simulink model "ROBOTIC_ARM_sim_v0"  (R2024b)
settings: Solver=VariableStepAuto  StartTime=0.0  StopTime=5  RelTol=1e-3
model workspace: external: MATLAB File D:\Vaults\Mechatronic Systems Design Project\Arm\Control\robotic_arm_4dof_matlab\scripts\initalize_model.m (data not in the file)
undefined symbols (not defined in the file): cubes, sim_relative, smiData, v_b, X, Y, Z
libraries: sm_lib x75, nesl_utility x21
(part 1 of 2)
settings Model: Creator=Mohammed Hany  LastModifiedBy=Mohammed Hany

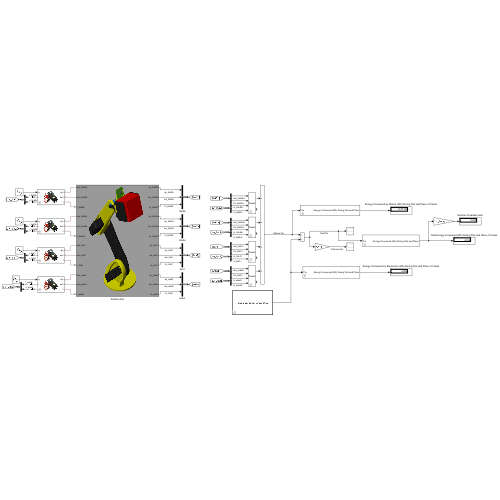
[thumbnail: Simulink's stored preview of the top-level diagram]
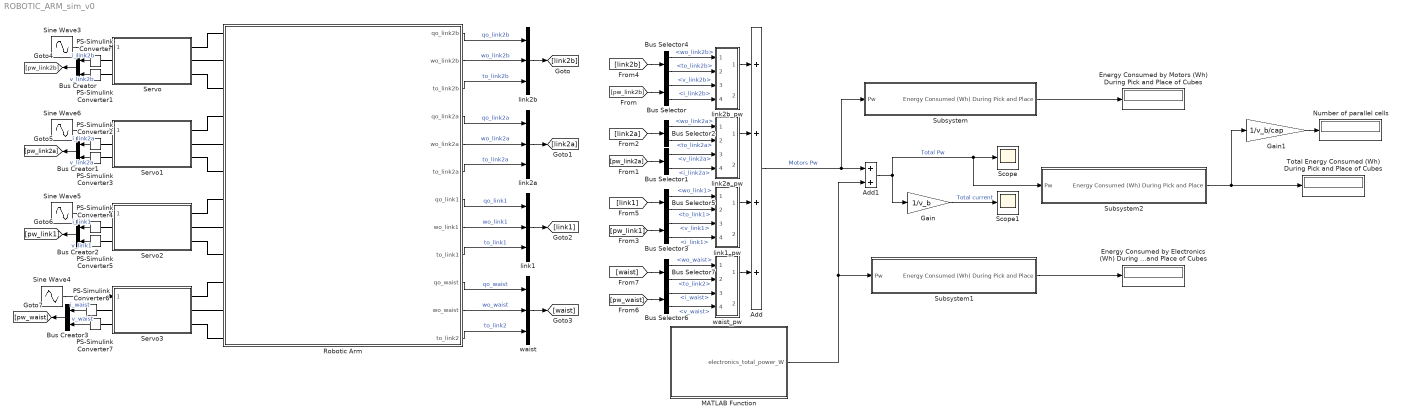
== system ROBOTIC_ARM_sim_v0 ==
  Add : Sum  Inputs=++++
  Add1 : Sum
  Bus Creator{,1..3} (4 alike) : BusCreator  Inputs=2
  Bus Selector : BusSelector  OutputSignals=v_link2b,i_link2b
  Bus Selector1 : BusSelector  OutputSignals=v_link2a,i_link2a
  Bus Selector2 : BusSelector  OutputSignals=wo_link2a,to_link2a
  Bus Selector3 : BusSelector  OutputSignals=v_link1,i_link1
  Bus Selector4 : BusSelector  OutputSignals=wo_link2b,to_link2b
  Bus Selector5 : BusSelector  OutputSignals=wo_link1,to_link1
  Bus Selector6 : BusSelector  OutputSignals=i_waist,v_waist
  Bus Selector7 : BusSelector  OutputSignals=wo_waist,to_link2
  Energy Consumed by Electronics (Wh) During Pick and Place of Cubes : Display
  Energy Consumed by Motors (Wh) During Pick and Place of Cubes : Display
  Gain : Gain  Gain=1/v_b
  Gain1 : Gain  Gain=1/v_b/cap
  MATLAB Function : MATLAB Function  TreatAsAtomicUnit=on
  Number of parallel cells : Display
  PS-Simulink Converter{,2,4,6} (4 alike) : nesl_utility/PS-Simulink Converter  PhysicalDomain=network_engine_domain  SubClassName=ps_output  LeftPortType=input  RightPortType=output  PseudoPeriodic=off  Frequencies=[]  VectorFormat=inherit  Unit=A  AffineConversion=off
  PS-Simulink Converter{1,3,5,7} (4 alike) : nesl_utility/PS-Simulink Converter  PhysicalDomain=network_engine_domain  SubClassName=ps_output  LeftPortType=input  RightPortType=output  PseudoPeriodic=off  Frequencies=[]  VectorFormat=inherit  Unit=V  AffineConversion=off
  Robotic Arm : Subsystem
      mask Display: image('isometric.png');
  Scope : Scope
  Scope1 : Scope
  Servo{,1..3} (4 alike) : Subsystem  ReferencedSubsystem=Servo  J=0 cm^2*g  La=12e-6 H  P_rated=4.2 W  V_i_noload=6 V  V_rated=6 V  i_noload=0.05 A  w_max=99 rpm  w_rated=71.43 rpm  ratio=1
  Sine Wave3 : Sin  Amplitude=55  Bias=30  SampleTime=0
  Sine Wave4 : Sin  Amplitude=180  SampleTime=0
  Sine Wave5 : Sin  Amplitude=100  Bias=-50  SampleTime=0
  Sine Wave6 : Sin  Amplitude=100  Bias=50  SampleTime=0
  Subsystem : Subsystem  mask{cubes=cubes}
      mask prompts: cubes "Number of cubes for pick and place"
  Subsystem1 : Subsystem  mask{cubes=cubes}
      mask prompts: cubes "Number of cubes for pick and place"
  Subsystem2 : Subsystem  mask{cubes=cubes}
      mask prompts: cubes "Number of cubes for pick and place"
  Total Energy Consumed (Wh) During Pick and Place of Cubes : Display
  link1 : BusCreator  Inputs=3
  link1_pw : Subsystem  ReferencedSubsystem=joint_power
  link2a : BusCreator  Inputs=3
  link2a_pw : Subsystem  ReferencedSubsystem=joint_power
  link2b : BusCreator  Inputs=3
  link2b_pw : Subsystem  ReferencedSubsystem=joint_power
  waist : BusCreator  Inputs=3
  waist_pw : Subsystem  ReferencedSubsystem=joint_power
  wires:
  Add/1 -> Subsystem/1(Pw), Add1/1  "Motors Pw"
  Subsystem1/1(Energy Consumed (Wh) During Pick and Place) -> Energy Consumed by Electronics (Wh) During Pick and Place of Cubes/1
  MATLAB Function/1(electronics_total_power_W) -> Add1/2, Subsystem1/1(Pw)
  Subsystem/1(Energy Consumed (Wh) During Pick and Place) -> Energy Consumed by Motors (Wh) During Pick and Place of Cubes/1
  Gain/1 -> Scope1/1  "Total current"
  Add1/1 -> Gain/1, Subsystem2/1(Pw), Scope/1  "Total Pw"
  Subsystem2/1(Energy Consumed (Wh) During Pick and Place) -> Gain1/1, Total Energy Consumed (Wh) During Pick and Place of Cubes/1
  Gain1/1 -> Number of parallel cells/1
  Sine Wave3/1 -> Servo/1
  Sine Wave6/1 -> Servo1/1
  Sine Wave5/1 -> Servo2/1
  Sine Wave4/1 -> Servo3/1
  Robotic Arm/3(to_link2b) -> link2b/3  "to_link2b"
  Robotic Arm/2(wo_link2b) -> link2b/2  "wo_link2b"
  Robotic Arm/1(qo_link2b) -> link2b/1  "qo_link2b"
  Robotic Arm/5(wo_link2a) -> link2a/2  "wo_link2a"
  Robotic Arm/4(qo_link2a) -> link2a/1  "qo_link2a"
  Robotic Arm/6(to_link2a) -> link2a/3  "to_link2a"
  Robotic Arm/8(wo_link1) -> link1/2  "wo_link1"
  Robotic Arm/7(qo_link1) -> link1/1  "qo_link1"
  Robotic Arm/9(to_link1) -> link1/3  "to_link1"
  Robotic Arm/11(wo_waist) -> waist/2  "wo_waist"
  Robotic Arm/10(qo_waist) -> waist/1  "qo_waist"
  Robotic Arm/12(to_link2) -> waist/3  "to_link2"
  link2b/1 -> [link2b]
  link2a/1 -> [link2a]
  link1/1 -> [link1]
  waist/1 -> [waist]
  PS-Simulink Converter/1 -> Bus Creator/1  "i_link2b"
  PS-Simulink Converter1/1 -> Bus Creator/2  "v_link2b"
  Bus Creator/1 -> [pw_link2b]
  PS-Simulink Converter3/1 -> Bus Creator1/2  "v_link2a"
  Bus Creator1/1 -> [pw_link2a]
  PS-Simulink Converter2/1 -> Bus Creator1/1  "i_link2a"
  PS-Simulink Converter4/1 -> Bus Creator2/1  "i_link1"
  PS-Simulink Converter5/1 -> Bus Creator2/2  "v_link1"
  Bus Creator2/1 -> [pw_link1]
  Bus Creator3/1 -> [pw_waist]
  PS-Simulink Converter7/1 -> Bus Creator3/2  "v_waist"
  PS-Simulink Converter6/1 -> Bus Creator3/1  "i_waist"
  [pw_link2b] -> Bus Selector/1
  link2b_pw/1 -> Add/1
  Bus Selector/1 -> link2b_pw/3  "<v_link2b>"
  Bus Selector/2 -> link2b_pw/4  "<i_link2b>"
  [link2b] -> Bus Selector4/1
  Bus Selector4/2 -> link2b_pw/2  "<to_link2b>"
  Bus Selector4/1 -> link2b_pw/1  "<wo_link2b>"
  [link2a] -> Bus Selector2/1
  [pw_link2a] -> Bus Selector1/1
  link2a_pw/1 -> Add/2
  Bus Selector2/1 -> link2a_pw/1  "<wo_link2a>"
  Bus Selector2/2 -> link2a_pw/2  "<to_link2a>"
  [link1] -> Bus Selector5/1
  [pw_link1] -> Bus Selector3/1
  link1_pw/1 -> Add/3
  Bus Selector1/1 -> link2a_pw/3  "<v_link2a>"
  Bus Selector1/2 -> link2a_pw/4  "<i_link2a>"
  Bus Selector5/1 -> link1_pw/1  "<wo_link1>"
  Bus Selector5/2 -> link1_pw/2  "<to_link1>"
  Bus Selector3/1 -> link1_pw/3  "<v_link1>"
  Bus Selector3/2 -> link1_pw/4  "<i_link1>"
  [pw_waist] -> Bus Selector6/1
  [waist] -> Bus Selector7/1
  waist_pw/1 -> Add/4
  Bus Selector7/1 -> waist_pw/1  "<wo_waist>"
  Bus Selector7/2 -> waist_pw/2  "<to_link2>"
  Bus Selector6/1 -> waist_pw/3  "<i_waist>"
  Bus Selector6/2 -> waist_pw/4  "<v_waist>"
  connections:
  Robotic Arm/LConn1 -- Servo/RConn1
  Robotic Arm/LConn2 -- Servo/RConn2
  Robotic Arm/LConn3 -- Servo/RConn3
  Servo1/RConn1 -- Robotic Arm/LConn4
  Robotic Arm/LConn5 -- Servo1/RConn2
  Robotic Arm/LConn6 -- Servo1/RConn3
  Robotic Arm/LConn7 -- Servo2/RConn1
  Robotic Arm/LConn8 -- Servo2/RConn2
  Robotic Arm/LConn9 -- Servo2/RConn3
  Robotic Arm/LConn10 -- Servo3/RConn1
  Robotic Arm/LConn11 -- Servo3/RConn2
  Robotic Arm/LConn12 -- Servo3/RConn3
  Servo/LConn1 -- PS-Simulink Converter/LConn1
  PS-Simulink Converter1/LConn1 -- Servo/LConn2
  Servo1/LConn1 -- PS-Simulink Converter2/LConn1
  Servo1/LConn2 -- PS-Simulink Converter3/LConn1
  Servo2/LConn1 -- PS-Simulink Converter4/LConn1
  Servo2/LConn2 -- PS-Simulink Converter5/LConn1
  Servo3/LConn1 -- PS-Simulink Converter6/LConn1
  PS-Simulink Converter7/LConn1 -- Servo3/LConn2

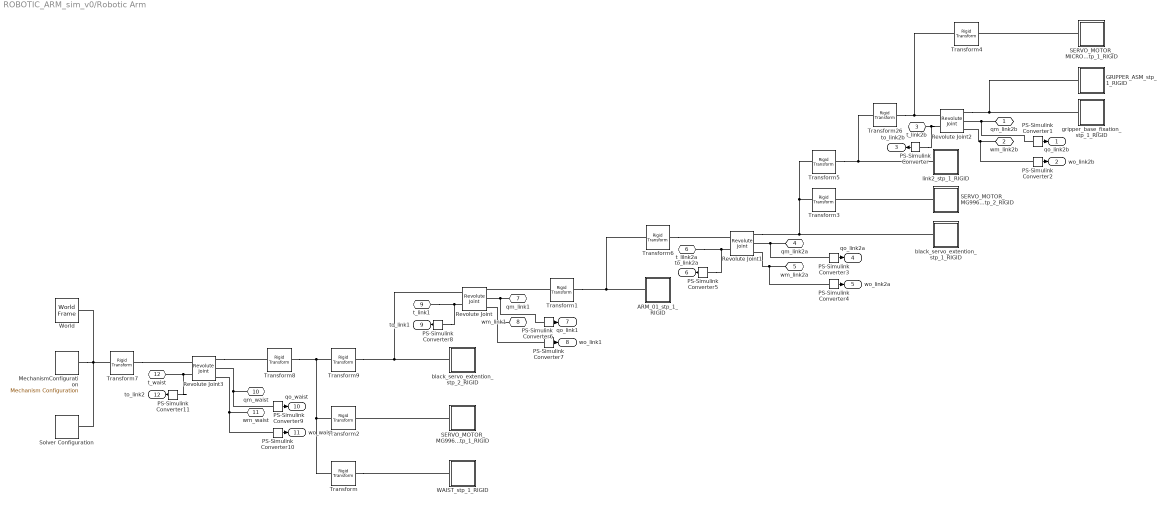
== system ROBOTIC_ARM_sim_v0/Robotic Arm ==
  ARM_01_stp_1_RIGID : Subsystem
  GRIPPER_ASM_stp_1_RIGID : Subsystem
  MechanismConfiguration : sm_lib/Utilities/Mechanism Configuration  UniformGravity=Constant  GravityVector=[0 0 0]  GravityVectorUnits=m/s^2  LinearizationDelta=0.001  JointModeTransitionNonlinearIterations=2
  PS-Simulink Converter{,5,8,11} (4 alike) : nesl_utility/PS-Simulink Converter  PhysicalDomain=network_engine_domain  SubClassName=ps_output  LeftPortType=input  RightPortType=output  PseudoPeriodic=off  Frequencies=[]  VectorFormat=inherit  Unit=N*m  AffineConversion=off
  PS-Simulink Converter{1,3,6,9} (4 alike) : nesl_utility/PS-Simulink Converter  PhysicalDomain=network_engine_domain  SubClassName=ps_output  LeftPortType=input  RightPortType=output  PseudoPeriodic=off  Frequencies=[]  VectorFormat=inherit  Unit=deg  AffineConversion=off
  PS-Simulink Converter{2,4,7,10} (4 alike) : nesl_utility/PS-Simulink Converter  PhysicalDomain=network_engine_domain  SubClassName=ps_output  LeftPortType=input  RightPortType=output  PseudoPeriodic=off  Frequencies=[]  VectorFormat=inherit  Unit=rpm  AffineConversion=off
  Revolute Joint{,1..3} (4 alike) : sm_lib/Joints/Revolute Joint  JointMode=Normal  CompositeWrenchDir=FollowerOnBase  CompositeWrenchFrame=BaseFrame  SenseConstraintForce=off  SenseConstraintTorque=off  SenseTotalForce=off  SenseTotalTorque=off  PositionTargetSpecify=off  PositionTargetPriority=High  PositionTargetValue=0  PositionTargetValueUnits=deg  VelocityTargetSpecify=off  VelocityTargetPriority=High  VelocityTargetValue=0  VelocityTargetValueUnits=deg/s  EquilibriumPosition=0  EquilibriumPositionUnits=deg  SpringStiffness=0  SpringStiffnessUnits=N*m/deg  DampingCoefficient=0  DampingCoefficientUnits=N*m/(deg/s)  LowerLimitSpecify=off  LowerLimitBound=-90  LowerLimitBoundUnits=deg  LowerLimitStiffness=1e4  LowerLimitStiffnessUnits=N*m/deg  LowerLimitDamping=10  LowerLimitDampingUnits=N*m/(deg/s)  LowerLimitTransitionRegionWidth=0.1  LowerLimitTransitionRegionWidthUnits=deg  UpperLimitSpecify=off  UpperLimitBound=90  UpperLimitBoundUnits=deg  UpperLimitStiffness=1e4  UpperLimitStiffnessUnits=N*m/deg  UpperLimitDamping=10  UpperLimitDampingUnits=N*m/(deg/s)  UpperLimitTransitionRegionWidth=0.1  UpperLimitTransitionRegionWidthUnits=deg  TorqueActuationMode=InputTorque  MotionActuationMode=ComputedMotion  SensePosition=on  SenseVelocity=on  SenseAcceleration=off  SenseTorqueForce=off  SenseLowerLimitTorqueForce=off  SenseUpperLimitTorqueForce=off
  SERVO_MOTOR_MG996R_stp_1_RIGID : Subsystem
  SERVO_MOTOR_MG996R_stp_2_RIGID : Subsystem
  SERVO_MOTOR_MICRO_9G_stp_1_RIGID : Subsystem
  Solver Configuration : nesl_utility/Solver Configuration  PhysicalDomain=network_engine_domain  SubClassName=solver  LeftPortType=input  RightPortType=generic  Tones=[]  Harmonics=[]  SimulateNoise=off  Profile=off  UseLocalSampling=off  EnableSwitchedLinearOptims=on  FrequencyDomain=off  UseCCode=off  RelTol=0.001  AbsTol=0.001  MinStep=1e-09  ToWorkspace=off  RevertToSquareIcSolve=off  NumHomotopyIterations=100  PhasorMode=off  PhasorModeNumHarmonics=1  ConsistencySolver=NEWTON_XTOL_AFTER_FTOL  IndexReductionMethod=DerivativeReplacement  DoDC=off  ResidualTolerance=1e-09  ConsistencyTolSource=GLOBAL  ConsistencyAbsTol=0.001  ConsistencyRelTol=0.001  ConsistencyTolFactor=0.001  UseLocalSolver=off  LocalSolverChoice=NE_BACKWARD_EULER_ADVANCER  ResolveIndetEquations=on  FunctionEvalNumThread=1  LocalSolverSampleTime=0.001  DoFixedCost=off  MaxNonlinIter=3  MaxModeIter=2  ComputeImpulses=off  ImpulseIterations=2  LinearAlgebra=auto  LinearAlgebraNumThread=0  EquationFormulation=NE_TIME_EF  DelaysMemoryBudget=1024  AutomaticFiltering=on  FilteringTimeConstant=0.001  PartitionStorageMethod=AS_NEEDED  PartitionMemoryBudget=1024  PartitionMethod=ROBUST  MultibodyUseLocalSolver=off  MultibodyLocalSolverChoice=ODE1  MultibodyLocalSolverSampleTime=0.001
  Transform : sm_lib/Frames and Transforms/Rigid Transform  RotationMethod=ArbitraryAxis  FollAlignAxisA=+X  BaseAlignAxisA=+Y  FollAlignAxisB=+Y  BaseAlignAxisB=+Z  RotationStandardAxis=+Z  RotationAngle=smiData.RigidTransform(25).angle  RotationAngleUnits=rad  RotationArbitraryAxis=smiData.RigidTransform(25).axis  RotationSequenceAxes=FollowerAxes  RotationSequence=XYX  RotationSequenceAngles=[0 0 0]  RotationSequenceAnglesUnits=deg  RotationMatrix=[1 0 0;0 1 0;0 0 1]  Quaternion=[1 0 0 0]  TranslationMethod=Cartesian  TranslationCartesianOffset=smiData.RigidTransform(25).translation  TranslationCartesianOffsetUnits=mm  TranslationStandardAxis=+Z  TranslationStandardOffset=0  TranslationStandardOffsetUnits=m  TranslationROffset=0  TranslationROffsetUnits=m  TranslationThetaOffset=0  TranslationThetaOffsetUnits=deg  TranslationZOffset=0  TranslationZOffsetUnits=m
  Transform1 : sm_lib/Frames and Transforms/Rigid Transform  RotationMethod=ArbitraryAxis  FollAlignAxisA=+X  BaseAlignAxisA=+Y  FollAlignAxisB=+Y  BaseAlignAxisB=+Z  RotationStandardAxis=+Z  RotationAngle=sim_relative(1).angle  RotationAngleUnits=rad  RotationArbitraryAxis=sim_relative(1).axis  RotationSequenceAxes=FollowerAxes  RotationSequence=XYX  RotationSequenceAngles=[0 0 0]  RotationSequenceAnglesUnits=deg  RotationMatrix=[1 0 0;0 1 0;0 0 1]  Quaternion=[1 0 0 0]  TranslationMethod=Cartesian  TranslationCartesianOffset=sim_relative(1).translation  TranslationCartesianOffsetUnits=mm  TranslationStandardAxis=+Z  TranslationStandardOffset=0  TranslationStandardOffsetUnits=m  TranslationROffset=0  TranslationROffsetUnits=m  TranslationThetaOffset=0  TranslationThetaOffsetUnits=deg  TranslationZOffset=0  TranslationZOffsetUnits=m
  Transform2 : sm_lib/Frames and Transforms/Rigid Transform  RotationMethod=ArbitraryAxis  FollAlignAxisA=+X  BaseAlignAxisA=+Y  FollAlignAxisB=+Y  BaseAlignAxisB=+Z  RotationStandardAxis=+Z  RotationAngle=smiData.RigidTransform(27).angle  RotationAngleUnits=rad  RotationArbitraryAxis=smiData.RigidTransform(27).axis  RotationSequenceAxes=FollowerAxes  RotationSequence=XYX  RotationSequenceAngles=[0 0 0]  RotationSequenceAnglesUnits=deg  RotationMatrix=[1 0 0;0 1 0;0 0 1]  Quaternion=[1 0 0 0]  TranslationMethod=Cartesian  TranslationCartesianOffset=smiData.RigidTransform(27).translation  TranslationCartesianOffsetUnits=mm  TranslationStandardAxis=+Z  TranslationStandardOffset=0  TranslationStandardOffsetUnits=m  TranslationROffset=0  TranslationROffsetUnits=m  TranslationThetaOffset=0  TranslationThetaOffsetUnits=deg  TranslationZOffset=0  TranslationZOffsetUnits=m
  Transform26 : sm_lib/Frames and Transforms/Rigid Transform  RotationMethod=ArbitraryAxis  FollAlignAxisA=+X  BaseAlignAxisA=+Y  FollAlignAxisB=+Y  BaseAlignAxisB=+Z  RotationStandardAxis=+Z  RotationAngle=sim_relative(5).angle  RotationAngleUnits=rad  RotationArbitraryAxis=sim_relative(5).axis  RotationSequenceAxes=FollowerAxes  RotationSequence=XYX  RotationSequenceAngles=[0 0 0]  RotationSequenceAnglesUnits=deg  RotationMatrix=[1 0 0;0 1 0;0 0 1]  Quaternion=[1 0 0 0]  TranslationMethod=Cartesian  TranslationCartesianOffset=sim_relative(5).translation  TranslationCartesianOffsetUnits=mm  TranslationStandardAxis=+Z  TranslationStandardOffset=0  TranslationStandardOffsetUnits=m  TranslationROffset=0  TranslationROffsetUnits=m  TranslationThetaOffset=0  TranslationThetaOffsetUnits=deg  TranslationZOffset=0  TranslationZOffsetUnits=m
  Transform3 : sm_lib/Frames and Transforms/Rigid Transform  RotationMethod=ArbitraryAxis  FollAlignAxisA=+X  BaseAlignAxisA=+Y  FollAlignAxisB=+Y  BaseAlignAxisB=+Z  RotationStandardAxis=+Z  RotationAngle=sim_relative(4).angle  RotationAngleUnits=rad  RotationArbitraryAxis=sim_relative(4).axis  RotationSequenceAxes=FollowerAxes  RotationSequence=XYX  RotationSequenceAngles=[0 0 0]  RotationSequenceAnglesUnits=deg  RotationMatrix=[1 0 0;0 1 0;0 0 1]  Quaternion=[1 0 0 0]  TranslationMethod=Cartesian  TranslationCartesianOffset=sim_relative(4).translation  TranslationCartesianOffsetUnits=mm  TranslationStandardAxis=+Z  TranslationStandardOffset=0  TranslationStandardOffsetUnits=m  TranslationROffset=0  TranslationROffsetUnits=m  TranslationThetaOffset=0  TranslationThetaOffsetUnits=deg  TranslationZOffset=0  TranslationZOffsetUnits=m
  Transform4 : sm_lib/Frames and Transforms/Rigid Transform  RotationMethod=ArbitraryAxis  FollAlignAxisA=+X  BaseAlignAxisA=+Y  FollAlignAxisB=+Y  BaseAlignAxisB=+Z  RotationStandardAxis=+Z  RotationAngle=sim_relative(8).angle  RotationAngleUnits=rad  RotationArbitraryAxis=sim_relative(8).axis  RotationSequenceAxes=FollowerAxes  RotationSequence=XYX  RotationSequenceAngles=[0 0 0]  RotationSequenceAnglesUnits=deg  RotationMatrix=[1 0 0;0 1 0;0 0 1]  Quaternion=[1 0 0 0]  TranslationMethod=Cartesian  TranslationCartesianOffset=sim_relative(8).translation  TranslationCartesianOffsetUnits=mm  TranslationStandardAxis=+Z  TranslationStandardOffset=0  TranslationStandardOffsetUnits=m  TranslationROffset=0  TranslationROffsetUnits=m  TranslationThetaOffset=0  TranslationThetaOffsetUnits=deg  TranslationZOffset=0  TranslationZOffsetUnits=m
  Transform5 : sm_lib/Frames and Transforms/Rigid Transform  RotationMethod=ArbitraryAxis  FollAlignAxisA=+X  BaseAlignAxisA=+Y  FollAlignAxisB=+Y  BaseAlignAxisB=+Z  RotationStandardAxis=+Z  RotationAngle=sim_relative(6).angle  RotationAngleUnits=rad  RotationArbitraryAxis=sim_relative(6).axis  RotationSequenceAxes=FollowerAxes  RotationSequence=XYX  RotationSequenceAngles=[0 0 0]  RotationSequenceAnglesUnits=deg  RotationMatrix=[1 0 0;0 1 0;0 0 1]  Quaternion=[1 0 0 0]  TranslationMethod=Cartesian  TranslationCartesianOffset=sim_relative(6).translation  TranslationCartesianOffsetUnits=mm  TranslationStandardAxis=+Z  TranslationStandardOffset=0  TranslationStandardOffsetUnits=m  TranslationROffset=0  TranslationROffsetUnits=m  TranslationThetaOffset=0  TranslationThetaOffsetUnits=deg  TranslationZOffset=0  TranslationZOffsetUnits=m
  Transform6 : sm_lib/Frames and Transforms/Rigid Transform  RotationMethod=ArbitraryAxis  FollAlignAxisA=+X  BaseAlignAxisA=+Y  FollAlignAxisB=+Y  BaseAlignAxisB=+Z  RotationStandardAxis=+Z  RotationAngle=sim_relative(3).angle  RotationAngleUnits=rad  RotationArbitraryAxis=sim_relative(3).axis  RotationSequenceAxes=FollowerAxes  RotationSequence=XYX  RotationSequenceAngles=[0 0 0]  RotationSequenceAnglesUnits=deg  RotationMatrix=[1 0 0;0 1 0;0 0 1]  Quaternion=[1 0 0 0]  TranslationMethod=Cartesian  TranslationCartesianOffset=sim_relative(3).translation  TranslationCartesianOffsetUnits=mm  TranslationStandardAxis=+Z  TranslationStandardOffset=0  TranslationStandardOffsetUnits=m  TranslationROffset=0  TranslationROffsetUnits=m  TranslationThetaOffset=0  TranslationThetaOffsetUnits=deg  TranslationZOffset=0  TranslationZOffsetUnits=m
  Transform7 : sm_lib/Frames and Transforms/Rigid Transform  RotationMethod=None  FollAlignAxisA=+X  BaseAlignAxisA=+Y  FollAlignAxisB=+Y  BaseAlignAxisB=+Z  RotationStandardAxis=+X  RotationAngle=pi/2  RotationAngleUnits=rad  RotationArbitraryAxis=smiData.RigidTransform(63).axis  RotationSequenceAxes=FollowerAxes  RotationSequence=XYX  RotationSequenceAngles=[0 0 0]  RotationSequenceAnglesUnits=deg  RotationMatrix=[1 0 0;0 1 0;0 0 1]  Quaternion=[1 0 0 0]  TranslationMethod=Cartesian  TranslationCartesianOffset=smiData.RigidTransform(63).translation  TranslationCartesianOffsetUnits=mm  TranslationStandardAxis=+Z  TranslationStandardOffset=0  TranslationStandardOffsetUnits=m  TranslationROffset=0  TranslationROffsetUnits=m  TranslationThetaOffset=0  TranslationThetaOffsetUnits=deg  TranslationZOffset=0  TranslationZOffsetUnits=m
  Transform8 : sm_lib/Frames and Transforms/Rigid Transform  RotationMethod=StandardAxis  FollAlignAxisA=+X  BaseAlignAxisA=+Y  FollAlignAxisB=+Y  BaseAlignAxisB=+Z  RotationStandardAxis=+X  RotationAngle=pi/2  RotationAngleUnits=rad  RotationArbitraryAxis=smiData.RigidTransform(63).axis  RotationSequenceAxes=FollowerAxes  RotationSequence=XYX  RotationSequenceAngles=[0 0 0]  RotationSequenceAnglesUnits=deg  RotationMatrix=[1 0 0;0 1 0;0 0 1]  Quaternion=[1 0 0 0]  TranslationMethod=Cartesian  TranslationCartesianOffset=smiData.RigidTransform(63).translation  TranslationCartesianOffsetUnits=mm  TranslationStandardAxis=+Z  TranslationStandardOffset=0  TranslationStandardOffsetUnits=m  TranslationROffset=0  TranslationROffsetUnits=m  TranslationThetaOffset=0  TranslationThetaOffsetUnits=deg  TranslationZOffset=0  TranslationZOffsetUnits=m
  Transform9 : sm_lib/Frames and Transforms/Rigid Transform  RotationMethod=ArbitraryAxis  FollAlignAxisA=+X  BaseAlignAxisA=+Y  FollAlignAxisB=+Y  BaseAlignAxisB=+Z  RotationStandardAxis=+Z  RotationAngle=smiData.RigidTransform(34).angle  RotationAngleUnits=rad  RotationArbitraryAxis=smiData.RigidTransform(34).axis  RotationSequenceAxes=FollowerAxes  RotationSequence=XYX  RotationSequenceAngles=[0 0 0]  RotationSequenceAnglesUnits=deg  RotationMatrix=[1 0 0;0 1 0;0 0 1]  Quaternion=[1 0 0 0]  TranslationMethod=Cartesian  TranslationCartesianOffset=smiData.RigidTransform(34).translation  TranslationCartesianOffsetUnits=mm  TranslationStandardAxis=+Z  TranslationStandardOffset=0  TranslationStandardOffsetUnits=m  TranslationROffset=0  TranslationROffsetUnits=m  TranslationThetaOffset=0  TranslationThetaOffsetUnits=deg  TranslationZOffset=0  TranslationZOffsetUnits=m
  WAIST_stp_1_RIGID : Subsystem
  World : sm_lib/Frames and Transforms/World Frame
  black_servo_extention_stp_1_RIGID : Subsystem
  black_servo_extention_stp_2_RIGID : Subsystem
  gripper_base_fixation_stp_1_RIGID : Subsystem
  link2_stp_1_RIGID : Subsystem
  qm_link2b : PMIOPort  Side=Left
  wm_link2b : PMIOPort  Port=2  Side=Left
  t_link2b : PMIOPort  Port=3  Side=Left
  qm_link2a : PMIOPort  Port=4  Side=Left
  wm_link2a : PMIOPort  Port=5  Side=Left
  t_lilnk2a : PMIOPort  Port=6  Side=Left
  qm_link1 : PMIOPort  Port=7  Side=Left
  wm_link1 : PMIOPort  Port=8  Side=Left
  t_link1 : PMIOPort  Port=9  Side=Left
  qm_waist : PMIOPort  Port=10  Side=Left
  wm_waist : PMIOPort  Port=11  Side=Left
  t_waist : PMIOPort  Port=12  Side=Left
  qo_link2b : Outport
  wo_link2b : Outport  Port=2
  to_link2b : Outport  Port=3
  qo_link2a : Outport  Port=4
  wo_link2a : Outport  Port=5
  to_link2a : Outport  Port=6
  qo_link1 : Outport  Port=7
  wo_link1 : Outport  Port=8
  to_link1 : Outport  Port=9
  qo_waist : Outport  Port=10
  wo_waist : Outport  Port=11
  to_link2 : Outport  Port=12
  wires:
  PS-Simulink Converter/1 -> to_link2b/1
  PS-Simulink Converter1/1 -> qo_link2b/1
  PS-Simulink Converter2/1 -> wo_link2b/1
  PS-Simulink Converter3/1 -> qo_link2a/1
  PS-Simulink Converter4/1 -> wo_link2a/1
  PS-Simulink Converter7/1 -> wo_link1/1
  PS-Simulink Converter6/1 -> qo_link1/1
  PS-Simulink Converter5/1 -> to_link2a/1
  PS-Simulink Converter8/1 -> to_link1/1
  PS-Simulink Converter9/1 -> qo_waist/1
  PS-Simulink Converter10/1 -> wo_waist/1
  PS-Simulink Converter11/1 -> to_link2/1
  connections:
  Transform/RConn1 -- WAIST_stp_1_RIGID/LConn1
  Transform9/LConn1 -- Transform2/LConn1 -- Transform/LConn1 -- Transform8/RConn1
  Transform9/RConn1 -- Revolute Joint/LConn1 -- black_servo_extention_stp_2_RIGID/LConn1
  SERVO_MOTOR_MG996R_stp_1_RIGID/LConn1 -- Transform2/RConn1
  Transform1/RConn1 -- Transform6/LConn1 -- ARM_01_stp_1_RIGID/LConn1
  Transform1/LConn1 -- Revolute Joint/RConn1
  Revolute Joint2/RConn1 -- GRIPPER_ASM_stp_1_RIGID/RConn1 -- gripper_base_fixation_stp_1_RIGID/LConn1
  SERVO_MOTOR_MG996R_stp_2_RIGID/LConn1 -- Transform3/RConn1
  Transform5/RConn1 -- Transform26/LConn1 -- link2_stp_1_RIGID/LConn1
  Transform6/RConn1 -- Revolute Joint1/LConn1
  Revolute Joint1/RConn1 -- Transform5/LConn1 -- Transform3/LConn1 -- black_servo_extention_stp_1_RIGID/LConn1
  Transform26/RConn1 -- Transform4/LConn1 -- Revolute Joint2/LConn1
  SERVO_MOTOR_MICRO_9G_stp_1_RIGID/LConn1 -- Transform4/RConn1
  World/RConn1 -- MechanismConfiguration/RConn1 -- Solver Configuration/RConn1 -- Transform7/LConn1
  Transform7/RConn1 -- Revolute Joint3/LConn1
  Revolute Joint3/LConn2 -- PS-Simulink Converter11/LConn1 -- t_waist/RConn1
  t_link2b/RConn1 -- PS-Simulink Converter/LConn1 -- Revolute Joint2/LConn2
  Revolute Joint3/RConn1 -- Transform8/LConn1
  wm_waist/RConn1 -- Revolute Joint3/RConn3 -- PS-Simulink Converter10/LConn1
  qm_waist/RConn1 -- PS-Simulink Converter9/LConn1 -- Revolute Joint3/RConn2
  t_lilnk2a/RConn1 -- PS-Simulink Converter5/LConn1 -- Revolute Joint1/LConn2
  qm_link2a/RConn1 -- PS-Simulink Converter3/LConn1 -- Revolute Joint1/RConn2
  wm_link2a/RConn1 -- PS-Simulink Converter4/LConn1 -- Revolute Joint1/RConn3
  wm_link2b/RConn1 -- PS-Simulink Converter2/LConn1 -- Revolute Joint2/RConn3
  qm_link2b/RConn1 -- PS-Simulink Converter1/LConn1 -- Revolute Joint2/RConn2
  t_link1/RConn1 -- PS-Simulink Converter8/LConn1 -- Revolute Joint/LConn2
  qm_link1/RConn1 -- PS-Simulink Converter6/LConn1 -- Revolute Joint/RConn2
  wm_link1/RConn1 -- Revolute Joint/RConn3 -- PS-Simulink Converter7/LConn1

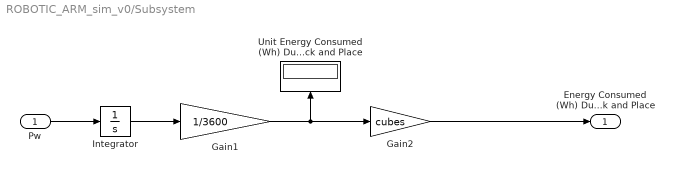
== system ROBOTIC_ARM_sim_v0/Subsystem ==
  Pw : Inport
  Gain1 : Gain  Gain=1/3600
  Gain2 : Gain  Gain=cubes
  Integrator : Integrator
  Unit Energy Consumed (Wh) During Pick and Place : Display
  Energy Consumed (Wh) During Pick and Place : Outport
  wires:
  Integrator/1 -> Gain1/1
  Gain1/1 -> Gain2/1, Unit Energy Consumed (Wh) During Pick and Place/1
  Gain2/1 -> Energy Consumed (Wh) During Pick and Place/1
  Pw/1 -> Integrator/1

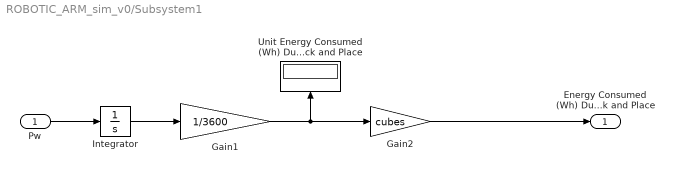
== system ROBOTIC_ARM_sim_v0/Subsystem1 ==
  Pw : Inport
  Gain1 : Gain  Gain=1/3600
  Gain2 : Gain  Gain=cubes
  Integrator : Integrator
  Unit Energy Consumed (Wh) During Pick and Place : Display
  Energy Consumed (Wh) During Pick and Place : Outport
  wires:
  Integrator/1 -> Gain1/1
  Gain1/1 -> Gain2/1, Unit Energy Consumed (Wh) During Pick and Place/1
  Gain2/1 -> Energy Consumed (Wh) During Pick and Place/1
  Pw/1 -> Integrator/1

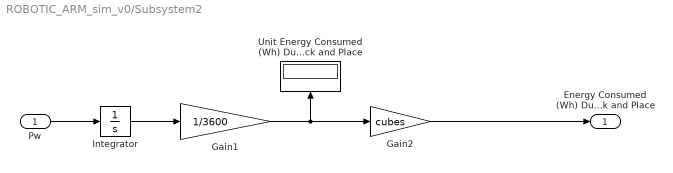
== system ROBOTIC_ARM_sim_v0/Subsystem2 ==
  Pw : Inport
  Gain1 : Gain  Gain=1/3600
  Gain2 : Gain  Gain=cubes
  Integrator : Integrator
  Unit Energy Consumed (Wh) During Pick and Place : Display
  Energy Consumed (Wh) During Pick and Place : Outport
  wires:
  Integrator/1 -> Gain1/1
  Gain1/1 -> Gain2/1, Unit Energy Consumed (Wh) During Pick and Place/1
  Gain2/1 -> Energy Consumed (Wh) During Pick and Place/1
  Pw/1 -> Integrator/1

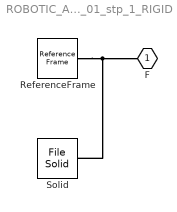
== system ROBOTIC_ARM_sim_v0/Robotic Arm/ARM_01_stp_1_RIGID ==
  ReferenceFrame : sm_lib/Frames and Transforms/Reference Frame
  Solid : sm_lib/Body Elements/File Solid  ExtGeomFileName=ARM 01.stp_Default_sldprt.STEP  UnitType=FromFile  ExtGeomFileUnits=m  StepReaderType=HEX  ExportConvexHullGeometry=off  InertiaType=Custom  BasedOnType=DensityFromFile  Density=1000  DensityUnits=kg/m^3  Mass=smiData.Solid(15).mass  MassUnits=kg  CenterOfMass=smiData.Solid(15).CoM  CenterOfMassUnits=mm  MomentsOfInertia=smiData.Solid(15).MoI  MomentsOfInertiaUnits=kg*mm^2  ProductsOfInertia=smiData.Solid(15).PoI  ProductsOfInertiaUnits=kg*mm^2  GraphicType=FromGeometry  MarkerShape=Sphere  MarkerSize=10  GraphicVisPropType=SimpleVisualProperties  GraphicDiffuseColor=[0.149 0.149 0.149]  GraphicOpacity=smiData.Solid(15).opacity  GraphicSpecularColor=[0.5 0.5 0.5 1.0]  GraphicAmbientColor=[0.15 0.15 0.15 1.0]  GraphicEmissiveColor=[0.0 0.0 0.0 1.0]  GraphicShininess=75  DoExposeReferenceFrame=on  SerializedFrames=<Frames/>
  F : PMIOPort  Side=Left
  connections:
  ReferenceFrame/RConn1 -- Solid/RConn1 -- F/RConn1

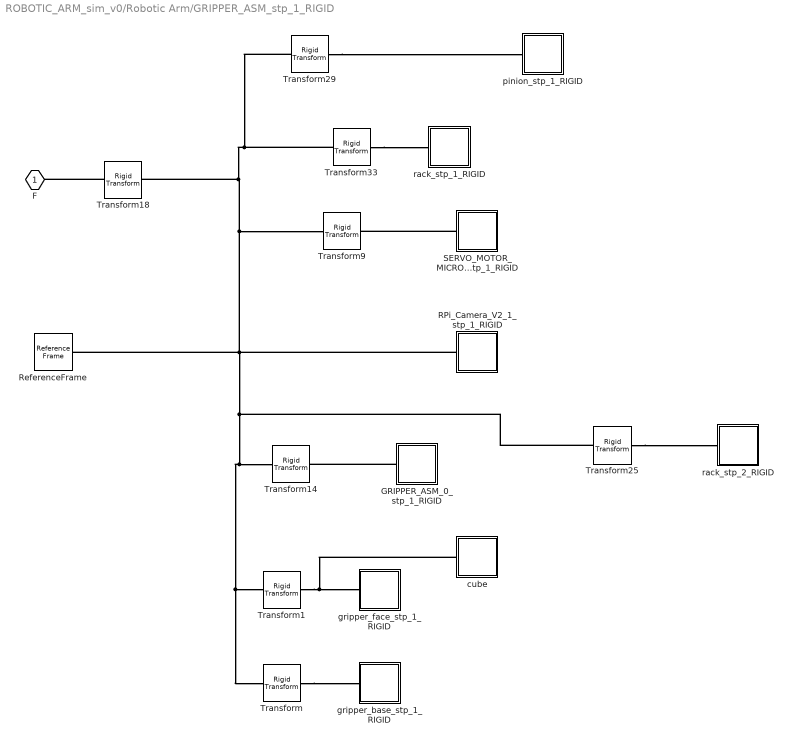
== system ROBOTIC_ARM_sim_v0/Robotic Arm/GRIPPER_ASM_stp_1_RIGID ==
  GRIPPER_ASM_0_stp_1_RIGID : Subsystem
  RPi_Camera_V2_1_stp_1_RIGID : Subsystem
  ReferenceFrame : sm_lib/Frames and Transforms/Reference Frame
  SERVO_MOTOR_MICRO_9G_stp_1_RIGID : Subsystem
  Transform : sm_lib/Frames and Transforms/Rigid Transform  RotationMethod=ArbitraryAxis  FollAlignAxisA=+X  BaseAlignAxisA=+Y  FollAlignAxisB=+Y  BaseAlignAxisB=+Z  RotationStandardAxis=+Z  RotationAngle=smiData.RigidTransform(1).angle  RotationAngleUnits=rad  RotationArbitraryAxis=smiData.RigidTransform(1).axis  RotationSequenceAxes=FollowerAxes  RotationSequence=XYX  RotationSequenceAngles=[0 0 0]  RotationSequenceAnglesUnits=deg  RotationMatrix=[1 0 0;0 1 0;0 0 1]  Quaternion=[1 0 0 0]  TranslationMethod=Cartesian  TranslationCartesianOffset=smiData.RigidTransform(1).translation  TranslationCartesianOffsetUnits=mm  TranslationStandardAxis=+Z  TranslationStandardOffset=0  TranslationStandardOffsetUnits=m  TranslationROffset=0  TranslationROffsetUnits=m  TranslationThetaOffset=0  TranslationThetaOffsetUnits=deg  TranslationZOffset=0  TranslationZOffsetUnits=m
  Transform1 : sm_lib/Frames and Transforms/Rigid Transform  RotationMethod=ArbitraryAxis  FollAlignAxisA=+X  BaseAlignAxisA=+Y  FollAlignAxisB=+Y  BaseAlignAxisB=+Z  RotationStandardAxis=+Z  RotationAngle=smiData.RigidTransform(7).angle  RotationAngleUnits=rad  RotationArbitraryAxis=smiData.RigidTransform(7).axis  RotationSequenceAxes=FollowerAxes  RotationSequence=XYX  RotationSequenceAngles=[0 0 0]  RotationSequenceAnglesUnits=deg  RotationMatrix=[1 0 0;0 1 0;0 0 1]  Quaternion=[1 0 0 0]  TranslationMethod=Cartesian  TranslationCartesianOffset=smiData.RigidTransform(7).translation  TranslationCartesianOffsetUnits=mm  TranslationStandardAxis=+Z  TranslationStandardOffset=0  TranslationStandardOffsetUnits=m  TranslationROffset=0  TranslationROffsetUnits=m  TranslationThetaOffset=0  TranslationThetaOffsetUnits=deg  TranslationZOffset=0  TranslationZOffsetUnits=m
  Transform14 : sm_lib/Frames and Transforms/Rigid Transform  RotationMethod=ArbitraryAxis  FollAlignAxisA=+X  BaseAlignAxisA=+Y  FollAlignAxisB=+Y  BaseAlignAxisB=+Z  RotationStandardAxis=+Z  RotationAngle=smiData.RigidTransform(20).angle  RotationAngleUnits=rad  RotationArbitraryAxis=smiData.RigidTransform(20).axis  RotationSequenceAxes=FollowerAxes  RotationSequence=XYX  RotationSequenceAngles=[0 0 0]  RotationSequenceAnglesUnits=deg  RotationMatrix=[1 0 0;0 1 0;0 0 1]  Quaternion=[1 0 0 0]  TranslationMethod=Cartesian  TranslationCartesianOffset=smiData.RigidTransform(20).translation  TranslationCartesianOffsetUnits=mm  TranslationStandardAxis=+Z  TranslationStandardOffset=0  TranslationStandardOffsetUnits=m  TranslationROffset=0  TranslationROffsetUnits=m  TranslationThetaOffset=0  TranslationThetaOffsetUnits=deg  TranslationZOffset=0  TranslationZOffsetUnits=m
  Transform18 : sm_lib/Frames and Transforms/Rigid Transform  RotationMethod=ArbitraryAxis  FollAlignAxisA=+X  BaseAlignAxisA=+Y  FollAlignAxisB=+Y  BaseAlignAxisB=+Z  RotationStandardAxis=+Z  RotationAngle=sim_relative(7).angle  RotationAngleUnits=rad  RotationArbitraryAxis=sim_relative(7).axis  RotationSequenceAxes=FollowerAxes  RotationSequence=XYX  RotationSequenceAngles=[0 0 0]  RotationSequenceAnglesUnits=deg  RotationMatrix=[1 0 0;0 1 0;0 0 1]  Quaternion=[1 0 0 0]  TranslationMethod=Cartesian  TranslationCartesianOffset=sim_relative(7).translation  TranslationCartesianOffsetUnits=mm  TranslationStandardAxis=+Z  TranslationStandardOffset=0  TranslationStandardOffsetUnits=m  TranslationROffset=0  TranslationROffsetUnits=m  TranslationThetaOffset=0  TranslationThetaOffsetUnits=deg  TranslationZOffset=0  TranslationZOffsetUnits=m
  Transform25 : sm_lib/Frames and Transforms/Rigid Transform  RotationMethod=ArbitraryAxis  FollAlignAxisA=+X  BaseAlignAxisA=+Y  FollAlignAxisB=+Y  BaseAlignAxisB=+Z  RotationStandardAxis=+Z  RotationAngle=sim_relative(10).angle  RotationAngleUnits=rad  RotationArbitraryAxis=sim_relative(10).axis  RotationSequenceAxes=FollowerAxes  RotationSequence=XYX  RotationSequenceAngles=[0 0 0]  RotationSequenceAnglesUnits=deg  RotationMatrix=[1 0 0;0 1 0;0 0 1]  Quaternion=[1 0 0 0]  TranslationMethod=Cartesian  TranslationCartesianOffset=sim_relative(10).translation  TranslationCartesianOffsetUnits=mm  TranslationStandardAxis=+Z  TranslationStandardOffset=0  TranslationStandardOffsetUnits=m  TranslationROffset=0  TranslationROffsetUnits=m  TranslationThetaOffset=0  TranslationThetaOffsetUnits=deg  TranslationZOffset=0  TranslationZOffsetUnits=m
  Transform29 : sm_lib/Frames and Transforms/Rigid Transform  RotationMethod=ArbitraryAxis  FollAlignAxisA=+X  BaseAlignAxisA=+Y  FollAlignAxisB=+Y  BaseAlignAxisB=+Z  RotationStandardAxis=+Z  RotationAngle=sim_relative(11).angle  RotationAngleUnits=rad  RotationArbitraryAxis=sim_relative(11).axis  RotationSequenceAxes=FollowerAxes  RotationSequence=XYX  RotationSequenceAngles=[0 0 0]  RotationSequenceAnglesUnits=deg  RotationMatrix=[1 0 0;0 1 0;0 0 1]  Quaternion=[1 0 0 0]  TranslationMethod=Cartesian  TranslationCartesianOffset=sim_relative(11).translation  TranslationCartesianOffsetUnits=mm  TranslationStandardAxis=+Z  TranslationStandardOffset=0  TranslationStandardOffsetUnits=m  TranslationROffset=0  TranslationROffsetUnits=m  TranslationThetaOffset=0  TranslationThetaOffsetUnits=deg  TranslationZOffset=0  TranslationZOffsetUnits=m
  Transform33 : sm_lib/Frames and Transforms/Rigid Transform  RotationMethod=ArbitraryAxis  FollAlignAxisA=+X  BaseAlignAxisA=+Y  FollAlignAxisB=+Y  BaseAlignAxisB=+Z  RotationStandardAxis=+Z  RotationAngle=sim_relative(9).angle  RotationAngleUnits=rad  RotationArbitraryAxis=sim_relative(9).axis  RotationSequenceAxes=FollowerAxes  RotationSequence=XYX  RotationSequenceAngles=[0 0 0]  RotationSequenceAnglesUnits=deg  RotationMatrix=[1 0 0;0 1 0;0 0 1]  Quaternion=[1 0 0 0]  TranslationMethod=Cartesian  TranslationCartesianOffset=sim_relative(9).translation  TranslationCartesianOffsetUnits=mm  TranslationStandardAxis=+Z  TranslationStandardOffset=0  TranslationStandardOffsetUnits=m  TranslationROffset=0  TranslationROffsetUnits=m  TranslationThetaOffset=0  TranslationThetaOffsetUnits=deg  TranslationZOffset=0  TranslationZOffsetUnits=m
  Transform9 : sm_lib/Frames and Transforms/Rigid Transform  RotationMethod=ArbitraryAxis  FollAlignAxisA=+X  BaseAlignAxisA=+Y  FollAlignAxisB=+Y  BaseAlignAxisB=+Z  RotationStandardAxis=+Z  RotationAngle=smiData.RigidTransform(15).angle  RotationAngleUnits=rad  RotationArbitraryAxis=smiData.RigidTransform(15).axis  RotationSequenceAxes=FollowerAxes  RotationSequence=XYX  RotationSequenceAngles=[0 0 0]  RotationSequenceAnglesUnits=deg  RotationMatrix=[1 0 0;0 1 0;0 0 1]  Quaternion=[1 0 0 0]  TranslationMethod=Cartesian  TranslationCartesianOffset=smiData.RigidTransform(15).translation  TranslationCartesianOffsetUnits=mm  TranslationStandardAxis=+Z  TranslationStandardOffset=0  TranslationStandardOffsetUnits=m  TranslationROffset=0  TranslationROffsetUnits=m  TranslationThetaOffset=0  TranslationThetaOffsetUnits=deg  TranslationZOffset=0  TranslationZOffsetUnits=m
  cube : Subsystem
  gripper_base_stp_1_RIGID : Subsystem
  gripper_face_stp_1_RIGID : Subsystem
  pinion_stp_1_RIGID : Subsystem
  rack_stp_1_RIGID : Subsystem
  rack_stp_2_RIGID : Subsystem
  F : PMIOPort  Side=Right
  connections:
  Transform/RConn1 -- gripper_base_stp_1_RIGID/LConn1
  Transform1/RConn1 -- cube/LConn1 -- gripper_face_stp_1_RIGID/LConn1
  GRIPPER_ASM_0_stp_1_RIGID/LConn1 -- Transform14/RConn1
  ReferenceFrame/RConn1 -- Transform29/LConn1 -- Transform33/LConn1 -- Transform18/RConn1 -- Transform9/LConn1 -- RPi_Camera_V2_1_stp_1_RIGID/RConn1 -- Transform25/LConn1 -- Transform14/LConn1 -- Transform/LConn1 -- Transform1/LConn1
  Transform18/LConn1 -- F/RConn1
  SERVO_MOTOR_MICRO_9G_stp_1_RIGID/LConn1 -- Transform9/RConn1
  Transform33/RConn1 -- rack_stp_1_RIGID/LConn1
  Transform25/RConn1 -- rack_stp_2_RIGID/LConn1
  Transform29/RConn1 -- pinion_stp_1_RIGID/LConn1

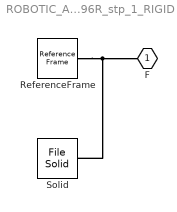
== system ROBOTIC_ARM_sim_v0/Robotic Arm/SERVO_MOTOR_MG996R_stp_1_RIGID ==
  ReferenceFrame : sm_lib/Frames and Transforms/Reference Frame
  Solid : sm_lib/Body Elements/File Solid  ExtGeomFileName=SERVO MOTOR MG996R.stp_Default_sldprt.STEP  UnitType=FromFile  ExtGeomFileUnits=m  StepReaderType=HEX  ExportConvexHullGeometry=off  InertiaType=Custom  BasedOnType=DensityFromFile  Density=1000  DensityUnits=kg/m^3  Mass=smiData.Solid(16).mass  MassUnits=kg  CenterOfMass=smiData.Solid(16).CoM  CenterOfMassUnits=mm  MomentsOfInertia=smiData.Solid(16).MoI  MomentsOfInertiaUnits=kg*mm^2  ProductsOfInertia=smiData.Solid(16).PoI  ProductsOfInertiaUnits=kg*mm^2  GraphicType=FromGeometry  MarkerShape=Sphere  MarkerSize=10  GraphicVisPropType=SimpleVisualProperties  GraphicDiffuseColor=[0.149 0.149 0.149]  GraphicOpacity=smiData.Solid(16).opacity  GraphicSpecularColor=[0.5 0.5 0.5 1.0]  GraphicAmbientColor=[0.15 0.15 0.15 1.0]  GraphicEmissiveColor=[0.0 0.0 0.0 1.0]  GraphicShininess=75  DoExposeReferenceFrame=on  SerializedFrames=<Frames/>
  F : PMIOPort  Side=Left
  connections:
  ReferenceFrame/RConn1 -- Solid/RConn1 -- F/RConn1

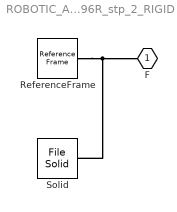
== system ROBOTIC_ARM_sim_v0/Robotic Arm/SERVO_MOTOR_MG996R_stp_2_RIGID ==
  ReferenceFrame : sm_lib/Frames and Transforms/Reference Frame
  Solid : sm_lib/Body Elements/File Solid  ExtGeomFileName=SERVO MOTOR MG996R.stp_Default_sldprt.STEP  UnitType=FromFile  ExtGeomFileUnits=m  StepReaderType=HEX  ExportConvexHullGeometry=off  InertiaType=Custom  BasedOnType=DensityFromFile  Density=1000  DensityUnits=kg/m^3  Mass=smiData.Solid(16).mass  MassUnits=kg  CenterOfMass=smiData.Solid(16).CoM  CenterOfMassUnits=mm  MomentsOfInertia=smiData.Solid(16).MoI  MomentsOfInertiaUnits=kg*mm^2  ProductsOfInertia=smiData.Solid(16).PoI  ProductsOfInertiaUnits=kg*mm^2  GraphicType=FromGeometry  MarkerShape=Sphere  MarkerSize=10  GraphicVisPropType=SimpleVisualProperties  GraphicDiffuseColor=[0.149 0.149 0.149]  GraphicOpacity=smiData.Solid(16).opacity  GraphicSpecularColor=[0.5 0.5 0.5 1.0]  GraphicAmbientColor=[0.15 0.15 0.15 1.0]  GraphicEmissiveColor=[0.0 0.0 0.0 1.0]  GraphicShininess=75  DoExposeReferenceFrame=on  SerializedFrames=<Frames/>
  F : PMIOPort  Side=Left
  connections:
  ReferenceFrame/RConn1 -- Solid/RConn1 -- F/RConn1

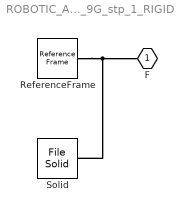
== system ROBOTIC_ARM_sim_v0/Robotic Arm/SERVO_MOTOR_MICRO_9G_stp_1_RIGID ==
  ReferenceFrame : sm_lib/Frames and Transforms/Reference Frame
  Solid : sm_lib/Body Elements/File Solid  ExtGeomFileName=SERVO MOTOR MICRO 9G.stp_Default_sldprt.STEP  UnitType=FromFile  ExtGeomFileUnits=m  StepReaderType=HEX  ExportConvexHullGeometry=off  InertiaType=Custom  BasedOnType=DensityFromFile  Density=1000  DensityUnits=kg/m^3  Mass=smiData.Solid(11).mass  MassUnits=kg  CenterOfMass=smiData.Solid(11).CoM  CenterOfMassUnits=mm  MomentsOfInertia=smiData.Solid(11).MoI  MomentsOfInertiaUnits=kg*mm^2  ProductsOfInertia=smiData.Solid(11).PoI  ProductsOfInertiaUnits=kg*mm^2  GraphicType=FromGeometry  MarkerShape=Sphere  MarkerSize=10  GraphicVisPropType=SimpleVisualProperties  GraphicDiffuseColor=[0.07451 0.6235 1]  GraphicOpacity=smiData.Solid(11).opacity  GraphicSpecularColor=[0.5 0.5 0.5 1.0]  GraphicAmbientColor=[0.15 0.15 0.15 1.0]  GraphicEmissiveColor=[0.0 0.0 0.0 1.0]  GraphicShininess=75  DoExposeReferenceFrame=on  SerializedFrames=<Frames/>
  F : PMIOPort  Side=Left
  connections:
  ReferenceFrame/RConn1 -- Solid/RConn1 -- F/RConn1

== system ROBOTIC_ARM_sim_v0/Robotic Arm/WAIST_stp_1_RIGID ==
  ReferenceFrame : sm_lib/Frames and Transforms/Reference Frame
  Solid : sm_lib/Body Elements/File Solid  ExtGeomFileName=WAIST.stp_Default_sldprt.STEP  UnitType=FromFile  ExtGeomFileUnits=m  StepReaderType=HEX  ExportConvexHullGeometry=off  InertiaType=Custom  BasedOnType=DensityFromFile  Density=1000  DensityUnits=kg/m^3  Mass=smiData.Solid(14).mass  MassUnits=kg  CenterOfMass=smiData.Solid(14).CoM  CenterOfMassUnits=mm  MomentsOfInertia=smiData.Solid(14).MoI  MomentsOfInertiaUnits=kg*mm^2  ProductsOfInertia=smiData.Solid(14).PoI  ProductsOfInertiaUnits=kg*mm^2  GraphicType=FromGeometry  MarkerShape=Sphere  MarkerSize=10  GraphicVisPropType=SimpleVisualProperties  GraphicDiffuseColor=[1 1 0]  GraphicOpacity=smiData.Solid(14).opacity  GraphicSpecularColor=[0.5 0.5 0.5 1.0]  GraphicAmbientColor=[0.15 0.15 0.15 1.0]  GraphicEmissiveColor=[0.0 0.0 0.0 1.0]  GraphicShininess=75  DoExposeReferenceFrame=on  SerializedFrames=<Frames/>
  F : PMIOPort  Side=Left
  connections:
  Solid/RConn1 -- ReferenceFrame/RConn1 -- F/RConn1

== system ROBOTIC_ARM_sim_v0/Robotic Arm/black_servo_extention_stp_1_RIGID ==
  ReferenceFrame : sm_lib/Frames and Transforms/Reference Frame
  Solid : sm_lib/Body Elements/File Solid  ExtGeomFileName=black servo extention.stp_Default_sldprt.STEP  UnitType=FromFile  ExtGeomFileUnits=m  StepReaderType=HEX  ExportConvexHullGeometry=off  InertiaType=Custom  BasedOnType=DensityFromFile  Density=1000  DensityUnits=kg/m^3  Mass=smiData.Solid(18).mass  MassUnits=kg  CenterOfMass=smiData.Solid(18).CoM  CenterOfMassUnits=mm  MomentsOfInertia=smiData.Solid(18).MoI  MomentsOfInertiaUnits=kg*mm^2  ProductsOfInertia=smiData.Solid(18).PoI  ProductsOfInertiaUnits=kg*mm^2  GraphicType=FromGeometry  MarkerShape=Sphere  MarkerSize=10  GraphicVisPropType=SimpleVisualProperties  GraphicDiffuseColor=[0.149 0.149 0.149]  GraphicOpacity=smiData.Solid(18).opacity  GraphicSpecularColor=[0.5 0.5 0.5 1.0]  GraphicAmbientColor=[0.15 0.15 0.15 1.0]  GraphicEmissiveColor=[0.0 0.0 0.0 1.0]  GraphicShininess=75  DoExposeReferenceFrame=on  SerializedFrames=<Frames/>
  F : PMIOPort  Side=Left
  connections:
  ReferenceFrame/RConn1 -- Solid/RConn1 -- F/RConn1

== system ROBOTIC_ARM_sim_v0/Robotic Arm/black_servo_extention_stp_2_RIGID ==
  ReferenceFrame : sm_lib/Frames and Transforms/Reference Frame
  Solid : sm_lib/Body Elements/File Solid  ExtGeomFileName=black servo extention.stp_Default_sldprt.STEP  UnitType=FromFile  ExtGeomFileUnits=m  StepReaderType=HEX  ExportConvexHullGeometry=off  InertiaType=Custom  BasedOnType=DensityFromFile  Density=1000  DensityUnits=kg/m^3  Mass=smiData.Solid(18).mass  MassUnits=kg  CenterOfMass=smiData.Solid(18).CoM  CenterOfMassUnits=mm  MomentsOfInertia=smiData.Solid(18).MoI  MomentsOfInertiaUnits=kg*mm^2  ProductsOfInertia=smiData.Solid(18).PoI  ProductsOfInertiaUnits=kg*mm^2  GraphicType=FromGeometry  MarkerShape=Sphere  MarkerSize=10  GraphicVisPropType=SimpleVisualProperties  GraphicDiffuseColor=[0.149 0.149 0.149]  GraphicOpacity=smiData.Solid(18).opacity  GraphicSpecularColor=[0.5 0.5 0.5 1.0]  GraphicAmbientColor=[0.15 0.15 0.15 1.0]  GraphicEmissiveColor=[0.0 0.0 0.0 1.0]  GraphicShininess=75  DoExposeReferenceFrame=on  SerializedFrames=<Frames/>
  F : PMIOPort  Side=Left
  connections:
  ReferenceFrame/RConn1 -- Solid/RConn1 -- F/RConn1

== system ROBOTIC_ARM_sim_v0/Robotic Arm/gripper_base_fixation_stp_1_RIGID ==
  ReferenceFrame : sm_lib/Frames and Transforms/Reference Frame
  Solid : sm_lib/Body Elements/File Solid  ExtGeomFileName=gripper base fixation.stp_Default_sldprt.STEP  UnitType=FromFile  ExtGeomFileUnits=m  StepReaderType=HEX  ExportConvexHullGeometry=off  InertiaType=Custom  BasedOnType=DensityFromFile  Density=1000  DensityUnits=kg/m^3  Mass=smiData.Solid(22).mass  MassUnits=kg  CenterOfMass=smiData.Solid(22).CoM  CenterOfMassUnits=mm  MomentsOfInertia=smiData.Solid(22).MoI  MomentsOfInertiaUnits=kg*mm^2  ProductsOfInertia=smiData.Solid(22).PoI  ProductsOfInertiaUnits=kg*mm^2  GraphicType=FromGeometry  MarkerShape=Sphere  MarkerSize=10  GraphicVisPropType=SimpleVisualProperties  GraphicDiffuseColor=[0.149 0.149 0.149]  GraphicOpacity=smiData.Solid(22).opacity  GraphicSpecularColor=[0.5 0.5 0.5 1.0]  GraphicAmbientColor=[0.15 0.15 0.15 1.0]  GraphicEmissiveColor=[0.0 0.0 0.0 1.0]  GraphicShininess=75  DoExposeReferenceFrame=on  SerializedFrames=<Frames/>
  F : PMIOPort  Side=Left
  connections:
  ReferenceFrame/RConn1 -- Solid/RConn1 -- F/RConn1

== system ROBOTIC_ARM_sim_v0/Robotic Arm/link2_stp_1_RIGID ==
  ReferenceFrame : sm_lib/Frames and Transforms/Reference Frame
  Solid : sm_lib/Body Elements/File Solid  ExtGeomFileName=link2.stp_Default_sldprt.STEP  UnitType=FromFile  ExtGeomFileUnits=m  StepReaderType=HEX  ExportConvexHullGeometry=off  InertiaType=Custom  BasedOnType=DensityFromFile  Density=1000  DensityUnits=kg/m^3  Mass=smiData.Solid(17).mass  MassUnits=kg  CenterOfMass=smiData.Solid(17).CoM  CenterOfMassUnits=mm  MomentsOfInertia=smiData.Solid(17).MoI  MomentsOfInertiaUnits=kg*mm^2  ProductsOfInertia=smiData.Solid(17).PoI  ProductsOfInertiaUnits=kg*mm^2  GraphicType=FromGeometry  MarkerShape=Sphere  MarkerSize=10  GraphicVisPropType=SimpleVisualProperties  GraphicDiffuseColor=[1 1 0]  GraphicOpacity=smiData.Solid(17).opacity  GraphicSpecularColor=[0.5 0.5 0.5 1.0]  GraphicAmbientColor=[0.15 0.15 0.15 1.0]  GraphicEmissiveColor=[0.0 0.0 0.0 1.0]  GraphicShininess=75  DoExposeReferenceFrame=on  SerializedFrames=<Frames/>
  F : PMIOPort  Side=Left
  connections:
  ReferenceFrame/RConn1 -- Solid/RConn1 -- F/RConn1

== system ROBOTIC_ARM_sim_v0/Robotic Arm/GRIPPER_ASM_stp_1_RIGID/GRIPPER_ASM_0_stp_1_RIGID ==
  ReferenceFrame : sm_lib/Frames and Transforms/Reference Frame
  Solid : sm_lib/Body Elements/File Solid  ExtGeomFileName=GRIPPER ASM-0.stp_Default_sldprt.STEP  UnitType=FromFile  ExtGeomFileUnits=m  StepReaderType=HEX  ExportConvexHullGeometry=off  InertiaType=Custom  BasedOnType=DensityFromFile  Density=1000  DensityUnits=kg/m^3  Mass=smiData.Solid(13).mass  MassUnits=kg  CenterOfMass=smiData.Solid(13).CoM  CenterOfMassUnits=mm  MomentsOfInertia=smiData.Solid(13).MoI  MomentsOfInertiaUnits=kg*mm^2  ProductsOfInertia=smiData.Solid(13).PoI  ProductsOfInertiaUnits=kg*mm^2  GraphicType=FromGeometry  MarkerShape=Sphere  MarkerSize=10  GraphicVisPropType=SimpleVisualProperties  GraphicDiffuseColor=smiData.Solid(13).color  GraphicOpacity=smiData.Solid(13).opacity  GraphicSpecularColor=[0.5 0.5 0.5 1.0]  GraphicAmbientColor=[0.15 0.15 0.15 1.0]  GraphicEmissiveColor=[0.0 0.0 0.0 1.0]  GraphicShininess=75  DoExposeReferenceFrame=on  SerializedFrames=<Frames/>
  F : PMIOPort  Side=Left
  connections:
  Solid/RConn1 -- ReferenceFrame/RConn1 -- F/RConn1
